simulink model "Q7_Simulation"  (R2022b)
settings: Solver=VariableStepAuto  StartTime=0.0  StopTime=25  RelTol=1e-3
undefined symbols (not defined in the file): A, B, C, K, K2
settings Model: Creator=amirz  LastModifiedBy=amirz

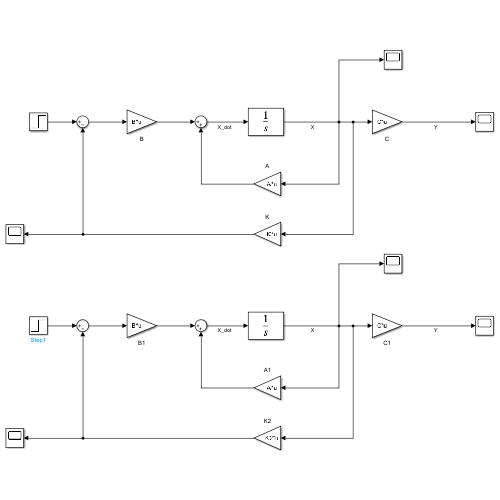
[thumbnail: Simulink's stored preview of the top-level diagram]
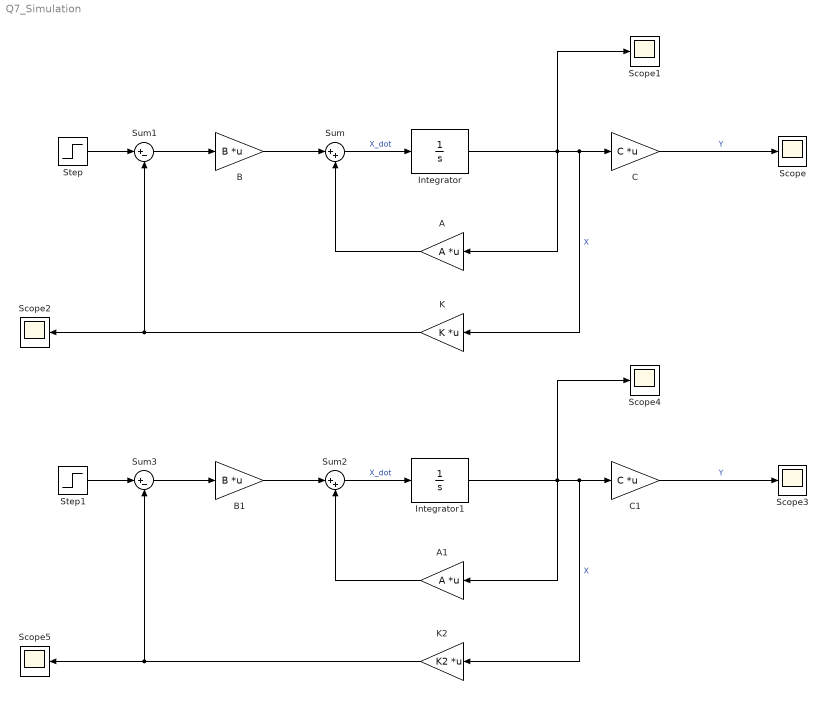
== system Q7_Simulation ==
  A : Gain  Gain=A  Multiplication=Matrix(K*u)
  A1 : Gain  Gain=A  Multiplication=Matrix(K*u)
  B : Gain  Gain=B  Multiplication=Matrix(K*u)
  B1 : Gain  Gain=B  Multiplication=Matrix(K*u)
  C : Gain  Gain=C  Multiplication=Matrix(K*u)
  C1 : Gain  Gain=C  Multiplication=Matrix(K*u)
  Integrator : Integrator
  Integrator1 : Integrator
  K : Gain  Gain=K  Multiplication=Matrix(K*u)
  K2 : Gain  Gain=K2  Multiplication=Matrix(K*u)
  Scope{,1..5} (6 alike) : Scope
  Step : Step  SampleTime=0
  Step1 : Step  SampleTime=0
  Sum : Sum  Inputs=|++
  Sum1 : Sum  Inputs=|+-
  Sum2 : Sum  Inputs=|++
  Sum3 : Sum  Inputs=|+-
  wires:
  Sum/1 -> Integrator/1  "X_dot"
  Integrator/1 -> Scope1/1, A/1, K/1, C/1  "X"
  A/1 -> Sum/2
  B/1 -> Sum/1
  Step/1 -> Sum1/1
  Sum1/1 -> B/1
  C/1 -> Scope/1  "Y"
  K/1 -> Scope2/1, Sum1/2
  Sum2/1 -> Integrator1/1  "X_dot"
  Sum3/1 -> B1/1
  C1/1 -> Scope3/1  "Y"
  Integrator1/1 -> Scope4/1, A1/1, K2/1, C1/1  "X"
  B1/1 -> Sum2/1
  Step1/1 -> Sum3/1
  K2/1 -> Scope5/1, Sum3/2
  A1/1 -> Sum2/2
